simulink model "DDSRFsinglephaseinverter"  (R2023b)
settings: Solver=VariableStepAuto  StartTime=0.0  StopTime=10  RelTol=1e-3
libraries: spsCurrentMeasurementLib x7, spsSeriesRLCBranchLib x7, spsAlphaBetaZerotodq0Lib x4, slpidlib x4, spsIGBTDiodeLib x4, spsVoltageMeasurementLib x4, spsabctoAlphaBetaZeroLib x2, spsdq0toAlphaBetaZeroLib x2, dspinverses x1, spsACVoltageSourceLib x1, spsBreakerLib x1, spsDCVoltageSourceLib x1
settings Model: Creator=Jia Yee Wong  LastModifiedBy=Jia Yee Wong
settings SFSimCC: SimCustomHeaderCode="#include \"ddsrfreferencegen.h\";"  SimUserSources=ddsrfreferencegen.c;

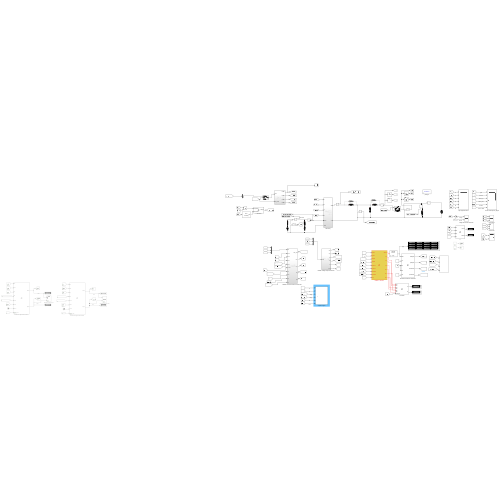
[thumbnail: Simulink's stored preview of the top-level diagram]
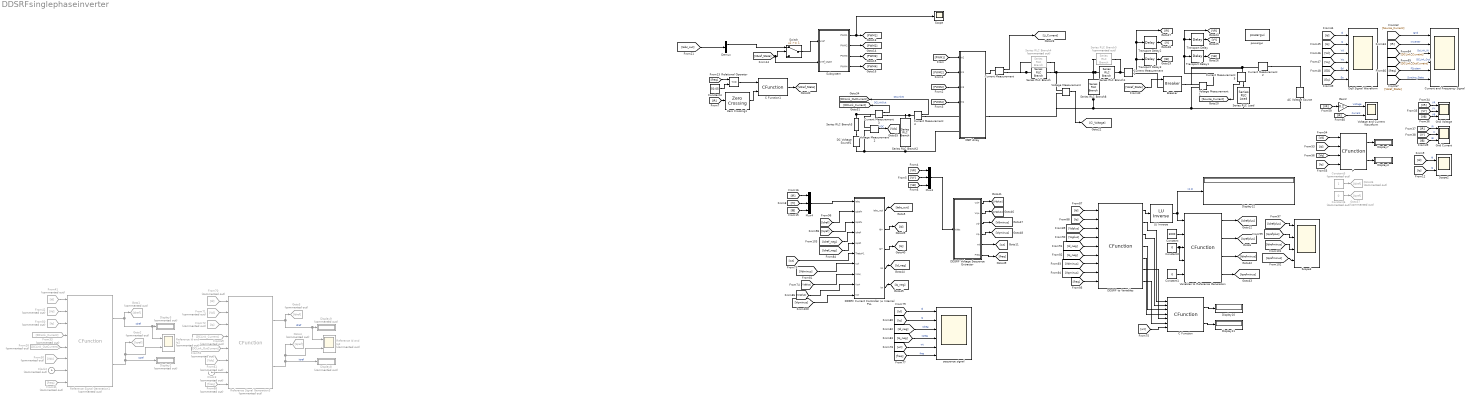
== system DDSRFsinglephaseinverter ==
  " LU Inverse" : dspinverses/ LU Inverse
  AC Voltage Source : spsACVoltageSourceLib/AC Voltage Source  Amplitude=340  Phase=0  Frequency=50  SampleTime=0  Measurements=None  BusType=PV  Pref=100  Qref=100  Qmin=-inf  Qmax=+inf
  Breaker : spsBreakerLib/Breaker  InitialState=0  SwitchingTimes="[1/60  5/60]"  External=on  BreakerResistance=0.00001  SnubberResistance=30  SnubberCapacitance=47e-9  Measurements=None  MoreParameters=on  NoBreakLoop=off
  C Function : CFunction  OutputCode=|
      | P= Po+Pc*cos(2*omegaT)+Ps*sin(2*omegaT);
      | Q= Qo+Qc*cos(2*omegaT)+Qs*sin(2*omegaT);
  C Function1 : CFunction  OutputCode=|  SampleTime=1/50000
      | if(Frequency == true && ZeroCross == 1){
      |     Output = 1;}
      | else if(Frequency == false){
      |         Output = 0;}
  Clock2 : Clock  Commented=on
  Clock3 : Clock  Commented=on
  Constant : Constant  Value=3000
  Constant1 : Constant  Value=0
  Constant2 : Constant  Value=0
  Constant4 : Constant  Value=50.05  SampleTime=1/50000
  Constant5 : Constant  Commented=on
  Constant6 : Constant  Commented=on  Value=0
  Current Measurement{,1..5} (6 alike) : spsCurrentMeasurementLib/Current Measurement  PhasorSimulation=off  OutputType=Complex  PSBequivalent=0
  Current and Frequency Signal : Scope  NumInputPorts=6
  DC Voltage Source1 : spsDCVoltageSourceLib/DC Voltage Source  Amplitude=400  Measurements=None
  DDSRF Current Controller /w Internal PLL : Subsystem
  DDSRF Voltage Sequence Extractor : Subsystem
  DDSRF to Variables : CFunction  OutputCode=|  SampleTime=1/50000
      | if(freq >49.9 && freq <50.1){
      |     Po=(Vdplus*Idplus+Vqplus*Iqplus+Vdminus*Idminus+Vqminus*Iqminus);
      |     Qo=(Vdplus*Idplus-Vqplus*Iqplus+Vdminus*Idminus-Vqminus*Iqminus);
      |     Pc=(Vdminus*Idplus+Vqminus*Iqplus+Vdplus*Iqminus+Vqplus*Iqminus);
      |     Ps=(Vqminus*Idplus-Vdminus*Iqplus-Vqplus*Idminus+Vdplus*Iqminus);
      |     Qc=(Vqminus*Idplus-Vdminus*Iqplus+Vdplus*Idminus-Vdplus*Iqminus);
      |     Qs=(-Vdminus*Idplus-Vqminus*Iqplus+Vdplus*Idminus+Vqplus*Iqminus);
      |     initializeMatrix(matref,Vdplus,Vqplus,Vdminus,Vqminus);
      |     
      |    
      |     }
  Demux : Demux  Outputs=3
  Display{4,7,10..12} (5 alike) : Display
  Display{2..3,8..9} (4 alike) : Display  Commented=on
  Dq0 Signal Waveform : Scope  NumInputPorts=6
  From26 : From  Commented=on  GotoTag=DCLink_OutCurrent
  From30 : From  Commented=on  GotoTag=Vdc
  From31 : From  Commented=on  GotoTag=freq
  From33 : From  Commented=on  GotoTag=DCLink_Current
  From41 : From  Commented=on  GotoTag=Id
  From42 : From  Commented=on  GotoTag=Vd
  From50 : From  Commented=on  GotoTag=Iq
  From51 : From  Commented=on  GotoTag=DCLink_OutCurrent
  From61 : From  Commented=on  GotoTag=Vdc
  From68 : From  Commented=on  GotoTag=freq
  From69 : From  Commented=on  GotoTag=DCLink_Current
  From70 : From  Commented=on  GotoTag=Id
  From71 : From  Commented=on  GotoTag=Vd
  From72 : From  Commented=on  GotoTag=Iq
  Gain2 : Gain  Gain=0.2
  Goto1 : Goto  Commented=on  GotoTag=Idref
  Goto2 : Goto  Commented=on  GotoTag=Iqref
  Goto3 : Goto  Commented=on  GotoTag=Idref
  Goto36 : Goto  Commented=on  GotoTag=Idref
  Goto37 : Goto  Commented=on  GotoTag=Iqref
  Goto4 : Goto  Commented=on  GotoTag=Iqref
  Grid Current : Scope  NumInputPorts=3
  Grid Voltage : Scope  NumInputPorts=3
  IGBT Array : Subsystem
  Mux3 : Mux  Inputs=3
  Mux4 : Mux  Inputs=3
  P : CFunction  OutputCode=|
      | PTotal = Id*Vd;
      | QTotal = Id*Vq-Vq*Id;
  Reference Id and Iq1 : Scope  Commented=on  NumInputPorts=2
  Reference Id and Iq2 : Scope  Commented=on  NumInputPorts=2
  Reference Signal Generation1 : CFunction  Commented=on  OutputCode=|  StartCode=|  SampleTime=1/50000
      OutputCode=|
      | if(Id!=PreviousId || Iq!=PreviousIq){
      |     if(ReferenceGenTrigger(Freq_PLL)){
      |         Idref=IdrefCalc(CLK,Vd,Iin,Iout, Vdc, Vdc);
      |   //Idref =1;
      |    Iqref=0;
      |    PreviousId=Id;
      |    PreviousIq=Iq;
      |    }
      |   
      | } else { Idref = 0; Iqref = 0;}
      StartCode=|
      | PreviousIq =0;
      | PreviousId =0;
  Reference Signal Generation3 : CFunction  Commented=on  OutputCode=|  StartCode=|  SampleTime=1/50000
      OutputCode=|
      | if(Id!=PreviousId || Iq!=PreviousIq){
      |     if(ReferenceGenTrigger(Freq_PLL)){
      |         Idref=IdrefCalc(CLK,Vd,Iin,Iout, Vdc, Vdc);
      |   //Idref =1;
      |    Iqref=0;
      |    PreviousId=Id;
      |    PreviousIq=Iq;
      |    }
      |   
      | } else { Idref = 0; Iqref = 0;}
      StartCode=|
      | PreviousIq =0;
      | PreviousId =0;
  Relational Operator : RelationalOperator  Operator=<=  OutDataTypeStr=boolean  RndMeth=Simplest  InputSameDT=off
  Scope : Scope
  Scope2 : Scope  NumInputPorts=2
  Scope3 : Scope  NumInputPorts=4
  Series RLC Branch : spsSeriesRLCBranchLib/Series RLC Branch  LConnTagsString=__new0  RConnTagsString=__new0  BranchType=L  Resistance=1  Inductance=20.4e-3  SetiL0=off  InitialCurrent=0  Capacitance=1e-6  Setx0=off  InitialVoltage=0  Measurements=None
  Series RLC Branch1 : spsSeriesRLCBranchLib/Series RLC Branch  LConnTagsString=__new0  RConnTagsString=__new0  BranchType=L  Resistance=1  Inductance=148.336e-6  SetiL0=off  InitialCurrent=0  Capacitance=1e-6  Setx0=off  InitialVoltage=0  Measurements=None
  Series RLC Branch2 : spsSeriesRLCBranchLib/Series RLC Branch  LConnTagsString=__new0  RConnTagsString=__new0  BranchType=RC  Resistance=1  Inductance=0  SetiL0=off  InitialCurrent=0  Capacitance=47e-3  Setx0=off  InitialVoltage=300  Measurements=None
  Series RLC Branch3 : spsSeriesRLCBranchLib/Series RLC Branch  LConnTagsString=__new0  RConnTagsString=__new0  BranchType=RL  Resistance=1  Inductance=0  SetiL0=off  InitialCurrent=0  Capacitance=1e-6  Setx0=off  InitialVoltage=0  Measurements=None
  Series RLC Branch4 : spsSeriesRLCBranchLib/Series RLC Branch  Commented=on  LConnTagsString=__new0  RConnTagsString=__new0  BranchType=R  Resistance=220  Inductance=20.4e-3  SetiL0=off  InitialCurrent=0  Capacitance=1e-6  Setx0=off  InitialVoltage=0  Measurements=None
  Series RLC Branch5 : spsSeriesRLCBranchLib/Series RLC Branch  Commented=on  LConnTagsString=__new0  RConnTagsString=__new0  BranchType=R  Resistance=220  Inductance=20.4e-3  SetiL0=off  InitialCurrent=0  Capacitance=1e-6  Setx0=off  InitialVoltage=0  Measurements=None
  Series RLC Branch8 : spsSeriesRLCBranchLib/Series RLC Branch  LConnTagsString=__new0  RConnTagsString=__new0  BranchType=RC  Resistance=120  Inductance=100e-6  SetiL0=off  InitialCurrent=0  Capacitance=5.526e-6  Setx0=off  InitialVoltage=0  Measurements=None
  Series RLC Load : spsSeriesRLCLoadLib/Series RLC Load  LConnTagsString=a  RConnTagsString=__new0  NominalVoltage=240  NominalFrequency=50  ActivePower=10e2  InductivePower=0  CapacitivePower=0  Setx0=off  InitialVoltage=240  SetiL0=off  InitialCurrent=10  Measurements=None  LoadType=constant PQ
  Subsystem : Subsystem
  Switch : Switch  Threshold=1  SaturateOnIntegerOverflow=off  InputSameDT=off
  Transport Delay : TransportDelay  DelayTime=6.67e-3  BufferSize=4096
  Transport Delay1 : TransportDelay  DelayTime=13.34e-3  BufferSize=5120
  Transport Delay2 : TransportDelay  DelayTime=6.67e-3  BufferSize=4096
  Transport Delay3 : TransportDelay  DelayTime=13.34e-3  BufferSize=4096
  Variables to Reference Generation : CFunction  OutputCode=|
      | Idrefplus = mat[0][0] * Po + mat[0][1] * 0 + mat[0][2] * 0 + mat[0][3] * Qo;
      | Iqrefplus = mat[1][0] * Po + mat[1][1] * 0 + mat[1][2] * 0 + mat[1][3] * Qo;
      | Idrefminus = mat[2][0] * Po - mat[2][1] * 0 - mat[2][2] * 0 + mat[2][3] * Qo;
      | Iqrefminus = mat[3][0] * Po - mat[3][1] * 0 + mat[3][2] * 0 - mat[3][3] * Qo;
  Voltage Measurement : spsVoltageMeasurementLib/Voltage Measurement  PhasorSimulation=off  OutputType=Complex  PSBequivalent=0
  Voltage Measurement1 : spsVoltageMeasurementLib/Voltage Measurement  PhasorSimulation=off  OutputType=Complex  PSBequivalent=0
  Voltage Measurement2 : spsVoltageMeasurementLib/Voltage Measurement  PhasorSimulation=off  OutputType=Complex  PSBequivalent=0
  Voltage and Current Waveform : Scope  NumInputPorts=2
  Zero Crossing1 : dspsigops/Zero Crossing
  powergui : spspowerguiLib/powergui  Priority=1  SimulationMode=Continuous  SampleTime=50e-6  frequency=60  Iterations=50  frequencyindice=0  Pbase=100e6  ErrMax=1e-4  UnitsV=kV  UnitsW=MW  buscounter=0  FunctionMessages=off  echomessages=off  EnableUseOfTLC=off  CurrentSourceSwitches=off  DisableSnubberDevices=off  DisableRonSwitches=off  DisableVfSwitches=off  DisplayEquations=off  AutomaticDiscreteSolvers=off  SolverType=Tustin/Backward Euler (TBE)  Interpol=off  ExternalGateDelay=off  methode=off  Ts=100  x0status=blocks  SPID=on  SwTol=0  HookPort=off  NonlinearTolerance=1e-4  nMaxIteration=100  ContinueOnMaxIteration=off  RestoreLinks=warning  ResistiveCurrentMeasurement=off  Frange=[0:2:500]  Ylog=off  Xlog=on  ShowGrid=off  save=off  variable=ZData  structure=0  ZoomFFT=off  StartTime=0.0  cycles=1  DisplayStyle=1  fundamental=60  FreqAxis=off  MaxFrequency=1000  frequencyindicesteady=1  RmsSteady=1  display=off
  sequence signal : Scope  NumInputPorts=6
  wires:
  [IR] -> Voltage and Current Waveform/2  "Current"
  [Iq] -> P/4
  Subsystem/4(PWM4) -> [PWM4]
  Switch/1 -> Subsystem/1(Vref)
  Constant5/1 -> Goto36/1
  [Id] -> P/2
  Current Measurement3/1 -> [DCLink_Current]  "DCLinkOut"
  Transport Delay3/1 -> [IB]
  [VY] -> Grid Voltage/2  "VY"
  [IY] -> Grid Current/2  "IY"
  Subsystem/1(PWM1) -> Scope/1, [PWM1]
  [VR] -> Grid Voltage/1  "VR"
  Demux/1 -> Switch/1
  [freq] -> Relational Operator/1
  Constant4/1 -> Relational Operator/2
  [VB] -> Grid Voltage/3  "VB"
  Subsystem/2(PWM2) -> [PWM2]
  Current Measurement/1 -> [Li_Current]
  Transport Delay1/1 -> [VB]
  Transport Delay2/1 -> [IY]
  Transport Delay/1 -> [VY]
  [VAref_State] -> Breaker/1
  [VR] -> Gain2/1
  Relational Operator/1 -> C Function1/1
  [IR] -> Current and Frequency Signal/2  "Iinverter"
  [Id] -> Scope2/1  "Id"
  Constant6/1 -> Goto37/1
  [Vd] -> Dq0 Signal Waveform/3  "Vd"
  C Function1/1 -> [VAref_State]
  Zero Crossing1/1 -> C Function1/2
  Current Measurement4/1 -> [DCLink_OutCurrent]  "DCLinkIN"
  [IR] -> Zero Crossing1/1
  [Source_Current] -> Current and Frequency Signal/1  "Igrid"
  [VAref_State] -> Current and Frequency Signal/6  "Synchro_State"
  Voltage Measurement2/1 -> [Vdc]  "VDC"
  Current Measurement1/1 -> [IR], Transport Delay2/1, Transport Delay3/1
  Gain2/1 -> Voltage and Current Waveform/1  "Voltage"
  [Vq] -> Dq0 Signal Waveform/4  "Vq"
  Subsystem/3(PWM3) -> [PWM3]
  [IB] -> Grid Current/3  "IB"
  [DCLink_OutCurrent] -> Current and Frequency Signal/4  "DCLink_Out"
  [PWM2] -> IGBT Array/2(In1)
  [DCLink_Current] -> Current and Frequency Signal/3  "DcLink_IN"
  [PWM3] -> IGBT Array/3(In3)
  [ED] -> Dq0 Signal Waveform/5  "Ed"
  Voltage Measurement1/1 -> [VR], Transport Delay/1, Transport Delay1/1
  P/1 -> Display7/1
  [IR] -> Grid Current/1  "IR"
  [Vq] -> P/3
  [PWM1] -> IGBT Array/1(In2)
  [Vd] -> P/1
  P/2 -> Display4/1
  [PWM4] -> IGBT Array/4(In4)
  Voltage Measurement/1 -> [Ci_Voltage]
  Current Measurement5/1 -> [Source_Current]
  [freq] -> Current and Frequency Signal/5  "FSystem"
  [Id] -> Dq0 Signal Waveform/1  "Id"
  [Iq] -> Dq0 Signal Waveform/2  "Iq"
  [Eq] -> Dq0 Signal Waveform/6  "Eq"
  [Iq] -> Scope2/2  "Iq"
  [VAref_State] -> Subsystem/2(Vref_state), Switch/2
  Reference Signal Generation1/1 -> Reference Id and Iq1/1, Display3/1, Goto1/1  "Idref"
  From26/1 -> Reference Signal Generation1/5
  From42/1 -> Reference Signal Generation1/2
  From50/1 -> Reference Signal Generation1/3
  From31/1 -> Reference Signal Generation1/8
  Reference Signal Generation1/2 -> Reference Id and Iq1/2, Goto2/1, Display2/1  "Iqref"
  Clock2/1 -> Reference Signal Generation1/7
  From30/1 -> Reference Signal Generation1/6
  From33/1 -> Reference Signal Generation1/4
  From41/1 -> Reference Signal Generation1/1
  From70/1 -> Reference Signal Generation3/1
  Clock3/1 -> Reference Signal Generation3/7
  From69/1 -> Reference Signal Generation3/4
  Reference Signal Generation3/2 -> Reference Id and Iq2/2, Goto4/1, Display8/1  "Iqref"
  From68/1 -> Reference Signal Generation3/8
  From61/1 -> Reference Signal Generation3/6
  From72/1 -> Reference Signal Generation3/3
  From71/1 -> Reference Signal Generation3/2
  From51/1 -> Reference Signal Generation3/5
  Reference Signal Generation3/1 -> Reference Id and Iq2/1, Display9/1, Goto3/1  "Idref"
  DDSRF to Variables/2 -> C Function/1
  C Function/1 -> Display10/1
  DDSRF to Variables/3 -> C Function/2
  [Vdplus] -> DDSRF Current Controller /w Internal PLL/8(Vd+\)
  C Function/2 -> Display11/1
  " LU Inverse"/1 -> Variables to Reference Generation/1, Display12/1  "[4 4]"
  [Id] -> sequence signal/1  "Id"
  [Id_neg] -> sequence signal/3  "Idneg"
  DDSRF to Variables/6 -> C Function/5
  [wt] -> DDSRF Current Controller /w Internal PLL/6(Theta*1)
  Constant1/1 -> Variables to Reference Generation/5
  Constant/1 -> Variables to Reference Generation/2
  [wt] -> sequence signal/5  "wt"
  [Iq_neg] -> sequence signal/4  "iqneg"
  DDSRF Voltage Sequence Extractor/5(wt) -> [wt]
  [Iq] -> sequence signal/2  "Iq"
  [Vqplus] -> DDSRF Current Controller /w Internal PLL/9(Vq+)
  [Vdminus] -> DDSRF Current Controller /w Internal PLL/7(Vd-)
  [Iqrefplus] -> Scope3/2
  [Idref_neg] -> DDSRF Current Controller /w Internal PLL/5(Iqref-)
  Variables to Reference Generation/2 -> [Iqrefplus]
  Variables to Reference Generation/1 -> [Idrefplus]
  [Vdminus] -> DDSRF to Variables/7
  [Vqminus] -> DDSRF Current Controller /w Internal PLL/10(Vq-)
  DDSRF Voltage Sequence Extractor/3(Vd-) -> [Vdminus]
  [Id_neg] -> DDSRF to Variables/5
  [Iqref] -> DDSRF Current Controller /w Internal PLL/3(Iqref+)
  [Idrefplus] -> Scope3/1
  [wt] -> C Function/7
  DDSRF to Variables/5 -> C Function/4
  [Iq_neg] -> DDSRF to Variables/6
  [Idrefminus] -> Scope3/3
  [Vdplus] -> DDSRF to Variables/3
  DDSRF Voltage Sequence Extractor/4(Vq-) -> [Vqminus]
  DDSRF Current Controller /w Internal PLL/3(Iq+) -> [Iq]
  Variables to Reference Generation/4 -> [Iqrefminus]
  [freq] -> sequence signal/6  "freq"
  [Id] -> DDSRF to Variables/1
  DDSRF Voltage Sequence Extractor/6(Freq) -> [freq]
  [Vqminus] -> DDSRF to Variables/8
  DDSRF to Variables/1 -> " LU Inverse"/1
  [freq] -> DDSRF to Variables/9
  Variables to Reference Generation/3 -> [Idrefminus]
  [Iqrefminus] -> Scope3/4
  DDSRF to Variables/7 -> C Function/6
  [Vqplus] -> DDSRF to Variables/4
  DDSRF Voltage Sequence Extractor/2(Vq+) -> [Vqplus]
  [Iq] -> DDSRF to Variables/2
  DDSRF Voltage Sequence Extractor/1(Vd+) -> [Vdplus]
  DDSRF Current Controller /w Internal PLL/1(Iabc_out) -> [Iabc_out]
  DDSRF Current Controller /w Internal PLL/2(Id+) -> [Id]
  [Idref_neg] -> DDSRF Current Controller /w Internal PLL/4(Idref-)
  DDSRF Current Controller /w Internal PLL/5(Iq-) -> [Iq_neg]
  DDSRF to Variables/4 -> C Function/3
  [Idref] -> DDSRF Current Controller /w Internal PLL/2(Idref+)
  DDSRF Current Controller /w Internal PLL/4(Id-) -> [Id_neg]
  Mux3/1 -> DDSRF Voltage Sequence Extractor/1(Vabc)
  [VB] -> Mux3/3
  [VR] -> Mux3/1
  [VY] -> Mux3/2
  Mux4/1 -> DDSRF Current Controller /w Internal PLL/1(Iabc)
  [IY] -> Mux4/2
  [IB] -> Mux4/3
  [IR] -> Mux4/1
  [Iabc_out] -> Demux/1
  Constant2/1 -> Variables to Reference Generation/4, Variables to Reference Generation/3
  connections:
  Current Measurement4/LConn1 -- Current Measurement3/RConn1 -- Series RLC Branch2/LConn1
  Series RLC Branch8/RConn1 -- IGBT Array/RConn2 -- Voltage Measurement/LConn2 -- AC Voltage Source/LConn1 -- Series RLC Load/RConn1 -- Voltage Measurement1/LConn2
  Voltage Measurement2/LConn2 -- Series RLC Branch2/RConn1 -- IGBT Array/LConn2 -- DC Voltage Source1/LConn1
  Series RLC Branch1/LConn1 -- Series RLC Branch8/LConn1 -- Series RLC Branch5/LConn1 -- Voltage Measurement/LConn1 -- Series RLC Branch/RConn1 -- Series RLC Branch4/RConn1
  Series RLC Branch3/LConn1 -- Current Measurement3/LConn1 -- Voltage Measurement2/LConn1
  Current Measurement1/LConn1 -- Series RLC Branch5/RConn1 -- Series RLC Branch1/RConn1
  Current Measurement2/RConn1 -- Breaker/RConn1 -- Voltage Measurement1/LConn1 -- Current Measurement5/LConn1
  Series RLC Branch/LConn1 -- Current Measurement/RConn1 -- Series RLC Branch4/LConn1
  IGBT Array/RConn1 -- Current Measurement/LConn1
  Current Measurement4/RConn1 -- IGBT Array/LConn1
  Breaker/LConn1 -- Current Measurement1/RConn1
  Current Measurement2/LConn1 -- AC Voltage Source/RConn1
  Current Measurement5/RConn1 -- Series RLC Load/LConn1
  Series RLC Branch3/RConn1 -- DC Voltage Source1/RConn1

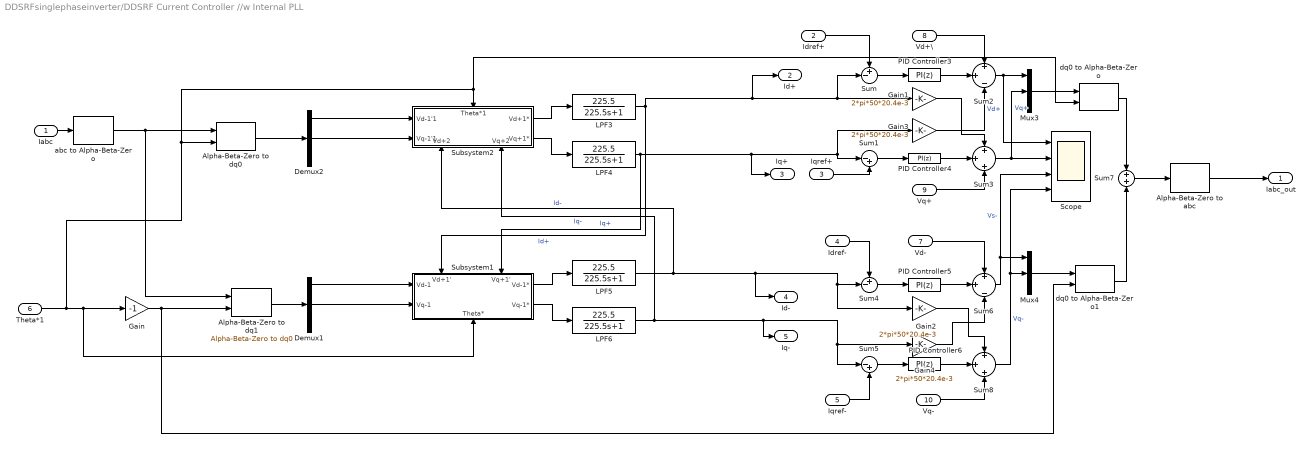
== system DDSRFsinglephaseinverter/DDSRF Current Controller //w Internal PLL ==
  Iabc : Inport
  Idref+ : Inport  Port=2
  Iqref+ : Inport  Port=3
  Idref- : Inport  Port=4
  Iqref- : Inport  Port=5
  Theta*1 : Inport  Port=6
  Vd- : Inport  Port=7
  Vd+\ : Inport  Port=8
  Vq+ : Inport  Port=9
  Vq- : Inport  Port=10
  Alpha-Beta-Zero to abc : spsAlphaBetaZerotoabcLib/Alpha-Beta-Zero to abc
      settings: LibrarySourceBlock=|
      | sps_lib/Control/Alpha-Beta-Zero
      | to abc
  Alpha-Beta-Zero to dq0 : spsAlphaBetaZerotodq0Lib/Alpha-Beta-Zero to dq0  Alignment=90 degrees behind phase A axis
  Alpha-Beta-Zero to dq1 : spsAlphaBetaZerotodq0Lib/Alpha-Beta-Zero to dq0  Alignment=90 degrees behind phase A axis
  Demux1 : Demux  Outputs=3
  Demux2 : Demux  Outputs=3
  Gain : Gain  Gain=-1
  Gain{1..4} (4 alike) : Gain  Gain=2*pi*50*20.4e-3
  LPF{3..6} (4 alike) : TransferFcn  Numerator=[225.5]  Denominator=[225.5 1]
  Mux3 : Mux  Inputs=3
  Mux4 : Mux  Inputs=3
  PID Controller{3..6} (4 alike) : slpidlib/PID Controller  Controller=PI  Form=Parallel  TimeDomain=Discrete-time  UseExternalTs=off  SampleTime=1/50000  IntegratorMethod=Forward Euler  FilterMethod=Forward Euler  ControllerParametersSource=internal  P=0.5  I=0.02  UseKiTs=off  D=0  N=100  UseFilter=on  TunerSelectOption=Transfer Function Based (PID Tuner App)  InitialConditionSource=internal  InitialConditionForIntegrator=0  InitialConditionForFilter=0  DifferentiatorICPrevScaledInput=0  ExternalReset=none  TrackingMode=off  Kt=1  LimitOutput=off  SatLimitsSource=internal  UpperSaturationLimit=inf  LowerSaturationLimit=-inf  LinearizeAsGain=on  AntiWindupMode=none  Kb=1  LimitIntegrator=off  UpperIntegratorSaturationLimit=inf  LowerIntegratorSaturationLimit=-inf  POutMin=[]  POutMax=[]  IOutMin=[]  IOutMax=[]  DOutMin=[]  DOutMax=[]  NOutMin=[]  NOutMax=[]  SumOutMin=[]  SumOutMax=[]  SaturationOutMin=[]  SaturationOutMax=[]  PParamMin=[]  PParamMax=[]  IParamMin=[]  IParamMax=[]  DParamMin=[]  DParamMax=[]  NParamMin=[]  NParamMax=[]  KbParamMin=[]  KbParamMax=[]  KtParamMin=[]  KtParamMax=[]  KbOutMin=[]  KbOutMax=[]  KtOutMin=[]  KtOutMax=[]  IntegratorOutMin=[]  IntegratorOutMax=[]  FilterOutMin=[]  FilterOutMax=[]  SumI1OutMin=[]  SumI1OutMax=[]  SumI2OutMin=[]  SumI2OutMax=[]  SumI3OutMin=[]  SumI3OutMax=[]  SumI4OutMin=[]  SumI4OutMax=[]  SumDOutMin=[]  SumDOutMax=[]  DifferentiatorOutMin=[]  DifferentiatorOutMax=[]  FilterDiffOutCoefMin=[]  FilterDiffOutCoefMax=[]  ReciprocalOutMin=[]  ReciprocalOutMax=[]  SumDenOutMin=[]  SumDenOutMax=[]  SumNumOutMin=[]  SumNumOutMax=[]  DivideOutMin=[]  DivideOutMax=[]  UdiffTsProdOutMin=[]  UdiffTsProdOutMax=[]  NTsProdOutMin=[]  NTsProdOutMax=[]  UintegralTsProdOutMin=[]  UintegralTsProdOutMax=[]  UngainTsProdOutMin=[]  UngainTsProdOutMax=[]  ClampingZeroOutDataTypeStr=Inherit: Inherit via back propagation  ClampingZeroOutMin=[]  ClampingZeroOutMax=[]  FilterDenConstantOutDataTypeStr=Inherit: Inherit via back propagation  FilterDenConstantOutMin=[]  FilterDenConstantOutMax=[]  PCopyOutDataTypeStr=Inherit: Inherit via back propagation  PCopyOutMin=[]  PCopyOutMax=[]  NCopyOutDataTypeStr=Inherit: Inherit via back propagation  NCopyOutMin=[]  NCopyOutMax=[]  IntegratorContinuousStateAttributes=''  IntegratorStateMustResolveToSignalObject=off  IntegratorRTWStateStorageClass=Auto  FilterContinuousStateAttributes=''  FilterStateMustResolveToSignalObject=off  FilterRTWStateStorageClass=Auto  ParallelPVariant=InternalParameters  IdealPVariant=Disabled  IVariant=InternalParameters  DVariant=Disabled  IntegratorVariant=Discrete  SatVariant=Disabled  AWVariant=Passthrough  PCopyVariant=Disabled  TRVariant=Disabled  FdbkBlocksVariant=Forward  IdealPFdbkVariant=Disabled  SatFdbkVariant=Disabled  DerivativeFilterVariant=Disabled  NVariant=Disabled  NCopyVariant=Disabled_SignalSpec  FilterICVariant=Disabled  IntegratorICVariant=InternalICs  ExternalResetVariant=Disabled  TRSumVariant=Passthrough  SumFdbkVariant=Disabled  SumVariant=Sum_PI  TsampFilterVariant=InternalTs  TsampNgainVariant=Passthrough  TsampIntegralVariant=Disabled_SignalSpec  ExternalSaturationOutDataTypeStr=Inherit: Same as second input
  Scope : Scope  NumInputPorts=4
  Subsystem1 : Subsystem
      settings: PortSchema="{\"entries\":[{\"content\":{\"sides\":[{\"content\":{\"connectorIds\":[\"In1\",\"In2\"]},\"type\":\"ConnectorPlacement.EquallySpacedRectSide\",\"uuid\":\"90520742-b67b-401b-a323-e780c78b1482\"},{\"content\":{\"connectorIds\":[\"Out1\",\"Out2\"],\"side\":\"RIGHT\"},\"type\":\"ConnectorPlacement.EquallySpacedRectSide\",\"uuid\":\"13b71677-6011-49b4-a8e2-8815d9fe4fc1\"},{\"content\":{\"connectorIds\":[\"In3\",\"In4\"],\"side\":\"TOP\"},\"type\":\"ConnectorPlacement.EquallySpacedRectSide\",\"uuid\":\"b0f32480-838e-4ed7-8c04-14ce7fe710af\"},{\"content\":{\"connectorIds\":[\"In5\"],\"side\":\"BOTTOM\"},\"type\":\"ConnectorPlacement.EquallySpacedRectSide\",\"uuid\":\"11e8df11-2f01-47a5-9567-d29a5352b573\"}]},\"type\":\"ConnectorPlacement.EquallySpacedConnector\",\"uuid\":\"d99c7ffd-2341-4980-bdb2-3a875f1b77ee\"}],\"packageUris\":[\"http://schema.mathworks.com/mf0/Connector/R2020b\"],\"version\":\"1.0\"}"
  Subsystem2 : Subsystem
      settings: PortSchema="{\"entries\":[{\"content\":{\"sides\":[{\"content\":{\"connectorIds\":[\"In1\",\"In2\"]},\"type\":\"ConnectorPlacement.EquallySpacedRectSide\",\"uuid\":\"90520742-b67b-401b-a323-e780c78b1482\"},{\"content\":{\"connectorIds\":[\"Out1\",\"Out2\"],\"side\":\"RIGHT\"},\"type\":\"ConnectorPlacement.EquallySpacedRectSide\",\"uuid\":\"13b71677-6011-49b4-a8e2-8815d9fe4fc1\"},{\"content\":{\"connectorIds\":[\"In3\"],\"side\":\"TOP\"},\"type\":\"ConnectorPlacement.EquallySpacedRectSide\",\"uuid\":\"b0f32480-838e-4ed7-8c04-14ce7fe710af\"},{\"content\":{\"connectorIds\":[\"In4\",\"In5\"],\"side\":\"BOTTOM\"},\"type\":\"ConnectorPlacement.EquallySpacedRectSide\",\"uuid\":\"7441e455-6112-4477-b61e-4bb135ec9e12\"}]},\"type\":\"ConnectorPlacement.EquallySpacedConnector\",\"uuid\":\"d99c7ffd-2341-4980-bdb2-3a875f1b77ee\"}],\"packageUris\":[\"http://schema.mathworks.com/mf0/Connector/R2020b\"],\"version\":\"1.0\"}"
  Sum : Sum  Inputs=+-|
  Sum1 : Sum  Inputs=|-+
  Sum2 : Sum  Inputs=+|+|-
  Sum3 : Sum  Inputs=+|+|+
  Sum4 : Sum  Inputs=+-|
  Sum5 : Sum  Inputs=|-+
  Sum6 : Sum  Inputs=+|+|-
  Sum7 : Sum  Inputs=+|+
  Sum8 : Sum  Inputs=+|+|+
  abc to Alpha-Beta-Zero : spsabctoAlphaBetaZeroLib/abc to Alpha-Beta-Zero
  dq0 to Alpha-Beta-Zero : spsdq0toAlphaBetaZeroLib/dq0 to Alpha-Beta-Zero  Alignment=90 degrees behind phase A axis
  dq0 to Alpha-Beta-Zero1 : spsdq0toAlphaBetaZeroLib/dq0 to Alpha-Beta-Zero  Alignment=90 degrees behind phase A axis
  Iabc_out : Outport
  Id+ : Outport  Port=2
  Iq+ : Outport  Port=3
  Id- : Outport  Port=4
  Iq- : Outport  Port=5
  wires:
  Mux3/1 -> dq0 to Alpha-Beta-Zero/1
  Gain2/1 -> Sum8/1
  Sum8/1 -> Scope/4, Mux4/2  "Vq-"
  LPF5/1 -> Gain2/1, Sum4/2, Id-/1, Subsystem2/4(Vd+2)  "Id-"
  Iabc/1 -> abc to Alpha-Beta-Zero/1
  Mux4/1 -> dq0 to Alpha-Beta-Zero1/1
  Idref-/1 -> Sum4/1
  Sum6/1 -> Scope/3, Mux4/1  "Vs-"
  LPF6/1 -> Iq-/1, Gain4/1, Sum5/1, Subsystem2/5(Vq+2)  "Iq-"
  Demux2/2 -> Subsystem2/2(Vq-1'1)
  Idref+/1 -> Sum/1
  Iqref+/1 -> Sum1/2
  dq0 to Alpha-Beta-Zero/1 -> Sum7/1
  LPF4/1 -> Subsystem1/4(Vq+1'), Iq+/1, Gain3/1, Sum1/1  "Iq+"
  Sum5/1 -> PID Controller6/1
  Sum/1 -> PID Controller3/1
  Subsystem2/1(Vd+1*) -> LPF3/1
  Demux2/1 -> Subsystem2/1(Vd-1'1)
  Subsystem1/2(Vq-1*) -> LPF6/1
  Sum1/1 -> PID Controller4/1
  dq0 to Alpha-Beta-Zero1/1 -> Sum7/2
  Iqref-/1 -> Sum5/2
  LPF3/1 -> Id+/1, Gain1/1, Sum/2, Subsystem1/3(Vd+1')  "Id+"
  Gain1/1 -> Sum3/1
  PID Controller6/1 -> Sum8/2
  Sum4/1 -> PID Controller5/1
  Sum3/1 -> Scope/2, Mux3/2  "Vq+"
  Subsystem1/1(Vd-1*) -> LPF5/1
  PID Controller4/1 -> Sum3/2
  Subsystem2/2(Vq+1*) -> LPF4/1
  Alpha-Beta-Zero to dq0/1 -> Demux2/1
  abc to Alpha-Beta-Zero/1 -> Alpha-Beta-Zero to dq0/1, Alpha-Beta-Zero to dq1/1
  Demux1/1 -> Subsystem1/1(Vd-1)
  Alpha-Beta-Zero to dq1/1 -> Demux1/1
  Gain/1 -> dq0 to Alpha-Beta-Zero1/2, Alpha-Beta-Zero to dq1/2
  Sum2/1 -> Scope/1, Mux3/1  "Vd+"
  Demux1/2 -> Subsystem1/2(Vq-1)
  Sum7/1 -> Alpha-Beta-Zero to abc/1
  Alpha-Beta-Zero to abc/1 -> Iabc_out/1
  Theta*1/1 -> Subsystem1/5(Theta*), Gain/1, Subsystem2/3(Theta*1), dq0 to Alpha-Beta-Zero/2, Alpha-Beta-Zero to dq0/2
  PID Controller3/1 -> Sum2/2
  Gain3/1 -> Sum2/3
  Gain4/1 -> Sum6/3
  PID Controller5/1 -> Sum6/2
  Vd-/1 -> Sum6/1
  Vd+\/1 -> Sum2/1
  Vq+/1 -> Sum3/3
  Vq-/1 -> Sum8/3

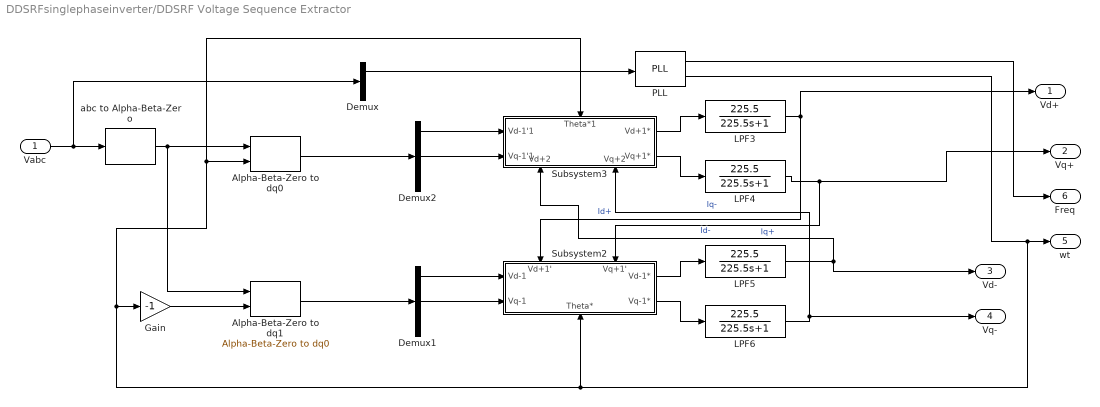
== system DDSRFsinglephaseinverter/DDSRF Voltage Sequence Extractor ==
  Vabc : Inport
  Alpha-Beta-Zero to dq0 : spsAlphaBetaZerotodq0Lib/Alpha-Beta-Zero to dq0  Alignment=90 degrees behind phase A axis
  Alpha-Beta-Zero to dq1 : spsAlphaBetaZerotodq0Lib/Alpha-Beta-Zero to dq0  Alignment=90 degrees behind phase A axis
  Demux : Demux  Outputs=3
  Demux1 : Demux  Outputs=3
  Demux2 : Demux  Outputs=3
  Gain : Gain  Gain=-1
  LPF{3..6} (4 alike) : TransferFcn  Numerator=[225.5]  Denominator=[225.5 1]
  PLL : spsPLLLib/PLL  Fmin=45  Par_Init=[0, 60]  ParK=[180, 3200, 1]  TcD=1e-4  MaxRateChangeFreq=12  FilterCutOffFreq=25  Ts=0  AGC=on
      settings: LibrarySourceBlock=sps_lib/Control/PLL
  Subsystem2 : Subsystem
      settings: PortSchema="{\"entries\":[{\"content\":{\"sides\":[{\"content\":{\"connectorIds\":[\"In1\",\"In2\"]},\"type\":\"ConnectorPlacement.EquallySpacedRectSide\",\"uuid\":\"90520742-b67b-401b-a323-e780c78b1482\"},{\"content\":{\"connectorIds\":[\"Out1\",\"Out2\"],\"side\":\"RIGHT\"},\"type\":\"ConnectorPlacement.EquallySpacedRectSide\",\"uuid\":\"13b71677-6011-49b4-a8e2-8815d9fe4fc1\"},{\"content\":{\"connectorIds\":[\"In3\",\"In4\"],\"side\":\"TOP\"},\"type\":\"ConnectorPlacement.EquallySpacedRectSide\",\"uuid\":\"b0f32480-838e-4ed7-8c04-14ce7fe710af\"},{\"content\":{\"connectorIds\":[\"In5\"],\"side\":\"BOTTOM\"},\"type\":\"ConnectorPlacement.EquallySpacedRectSide\",\"uuid\":\"11e8df11-2f01-47a5-9567-d29a5352b573\"}]},\"type\":\"ConnectorPlacement.EquallySpacedConnector\",\"uuid\":\"d99c7ffd-2341-4980-bdb2-3a875f1b77ee\"}],\"packageUris\":[\"http://schema.mathworks.com/mf0/Connector/R2020b\"],\"version\":\"1.0\"}"
  Subsystem3 : Subsystem
      settings: PortSchema="{\"entries\":[{\"content\":{\"sides\":[{\"content\":{\"connectorIds\":[\"In1\",\"In2\"]},\"type\":\"ConnectorPlacement.EquallySpacedRectSide\",\"uuid\":\"90520742-b67b-401b-a323-e780c78b1482\"},{\"content\":{\"connectorIds\":[\"Out1\",\"Out2\"],\"side\":\"RIGHT\"},\"type\":\"ConnectorPlacement.EquallySpacedRectSide\",\"uuid\":\"13b71677-6011-49b4-a8e2-8815d9fe4fc1\"},{\"content\":{\"connectorIds\":[\"In3\"],\"side\":\"TOP\"},\"type\":\"ConnectorPlacement.EquallySpacedRectSide\",\"uuid\":\"b0f32480-838e-4ed7-8c04-14ce7fe710af\"},{\"content\":{\"connectorIds\":[\"In4\",\"In5\"],\"side\":\"BOTTOM\"},\"type\":\"ConnectorPlacement.EquallySpacedRectSide\",\"uuid\":\"7441e455-6112-4477-b61e-4bb135ec9e12\"}]},\"type\":\"ConnectorPlacement.EquallySpacedConnector\",\"uuid\":\"d99c7ffd-2341-4980-bdb2-3a875f1b77ee\"}],\"packageUris\":[\"http://schema.mathworks.com/mf0/Connector/R2020b\"],\"version\":\"1.0\"}"
  abc to Alpha-Beta-Zero : spsabctoAlphaBetaZeroLib/abc to Alpha-Beta-Zero
  Vd+ : Outport
  Vq+ : Outport  Port=2
  Vd- : Outport  Port=3
  Vq- : Outport  Port=4
  wt : Outport  Port=5
  Freq : Outport  Port=6
  wires:
  Demux2/1 -> Subsystem3/1(Vd-1'1)
  Subsystem2/1(Vd-1*) -> LPF5/1
  LPF5/1 -> Vd-/1, Subsystem3/4(Vd+2)  "Id-"
  LPF4/1 -> Subsystem2/4(Vq+1'), Vq+/1  "Iq+"
  LPF6/1 -> Vq-/1, Subsystem3/5(Vq+2)  "Iq-"
  LPF3/1 -> Vd+/1, Subsystem2/3(Vd+1')  "Id+"
  Subsystem2/2(Vq-1*) -> LPF6/1
  Demux2/2 -> Subsystem3/2(Vq-1'1)
  Alpha-Beta-Zero to dq0/1 -> Demux2/1
  abc to Alpha-Beta-Zero/1 -> Alpha-Beta-Zero to dq1/1, Alpha-Beta-Zero to dq0/1
  Alpha-Beta-Zero to dq1/1 -> Demux1/1
  Demux1/1 -> Subsystem2/1(Vd-1)
  Demux1/2 -> Subsystem2/2(Vq-1)
  Gain/1 -> Alpha-Beta-Zero to dq1/2
  Vabc/1 -> Demux/1, abc to Alpha-Beta-Zero/1
  Subsystem3/1(Vd+1*) -> LPF3/1
  Subsystem3/2(Vq+1*) -> LPF4/1
  Demux/1 -> PLL/1
  PLL/2 -> Subsystem2/5(Theta*), Subsystem3/3(Theta*1), Alpha-Beta-Zero to dq0/2, Gain/1, wt/1
  PLL/1 -> Freq/1

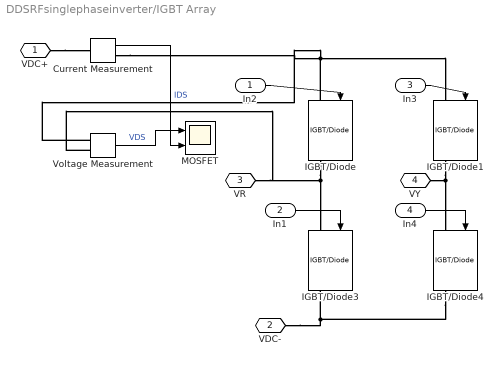
== system DDSRFsinglephaseinverter/IGBT Array ==
  In2 : Inport
  In1 : Inport  Port=2
  In3 : Inport  Port=3
  In4 : Inport  Port=4
  Current Measurement : spsCurrentMeasurementLib/Current Measurement  PhasorSimulation=off  OutputType=Complex  PSBequivalent=0
  IGBT/Diode{,1,3..4} (4 alike) : spsIGBTDiodeLib/IGBT//Diode  Ron=1e-3  Rs=1e5  Cs=inf  Measurements=on
  MOSFET : Scope  NumInputPorts=2
  Voltage Measurement : spsVoltageMeasurementLib/Voltage Measurement  PhasorSimulation=off  OutputType=Complex  PSBequivalent=0
  VDC+ : PMIOPort  Side=Left
  VDC- : PMIOPort  Port=2  Side=Left
  VR : PMIOPort  Port=3  Side=Right
  VY : PMIOPort  Port=4  Side=Right
  wires:
  In1/1 -> IGBT/Diode3/1
  In4/1 -> IGBT/Diode4/1
  In3/1 -> IGBT/Diode1/1
  In2/1 -> IGBT/Diode/1
  Voltage Measurement/1 -> MOSFET/1  "VDS"
  Current Measurement/1 -> MOSFET/2  "IDS"
  connections:
  IGBT/Diode4/RConn1 -- VDC-/RConn1 -- IGBT/Diode3/RConn1
  IGBT/Diode/RConn1 -- Voltage Measurement/LConn2 -- VR/RConn1 -- IGBT/Diode3/LConn1
  IGBT/Diode1/RConn1 -- VY/RConn1 -- IGBT/Diode4/LConn1
  IGBT/Diode/LConn1 -- Current Measurement/RConn1 -- Voltage Measurement/LConn1 -- IGBT/Diode1/LConn1
  VDC+/RConn1 -- Current Measurement/LConn1

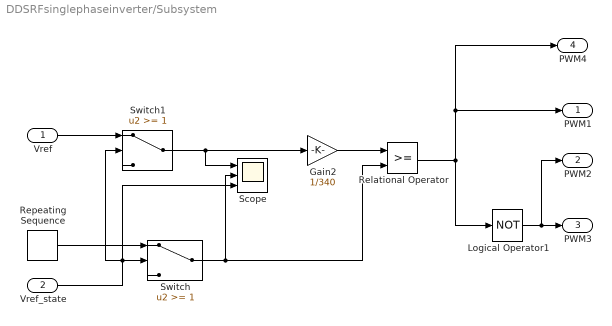
== system DDSRFsinglephaseinverter/Subsystem ==
  Vref : Inport
  Vref_state : Inport  Port=2
  Gain2 : Gain  Gain=1/340
  Logical Operator1 : Logic  Operator=NOT  AllPortsSameDT=off  OutDataTypeStr=boolean
  Relational Operator : RelationalOperator  OutDataTypeStr=boolean  RndMeth=Simplest  InputSameDT=off
  Repeating Sequence : simulink/Sources/Repeating Sequence  rep_seq_t=[0 0.00005 0.0001]  rep_seq_y=[-1 1 -1]
  Scope : Scope  NumInputPorts=3
  Switch : Switch  Threshold=1  SaturateOnIntegerOverflow=off  InputSameDT=off
  Switch1 : Switch  Threshold=1  SaturateOnIntegerOverflow=off  InputSameDT=off
  PWM1 : Outport
  PWM2 : Outport  Port=2
  PWM3 : Outport  Port=3
  PWM4 : Outport  Port=4
  wires:
  Gain2/1 -> Relational Operator/1
  Relational Operator/1 -> Logical Operator1/1, PWM1/1, PWM4/1
  Logical Operator1/1 -> PWM2/1, PWM3/1
  Repeating Sequence/1 -> Switch/1
  Switch/1 -> Scope/2, Relational Operator/2
  Vref_state/1 -> Scope/3, Switch1/2, Switch/2
  Switch1/1 -> Gain2/1, Scope/1
  Vref/1 -> Switch1/1

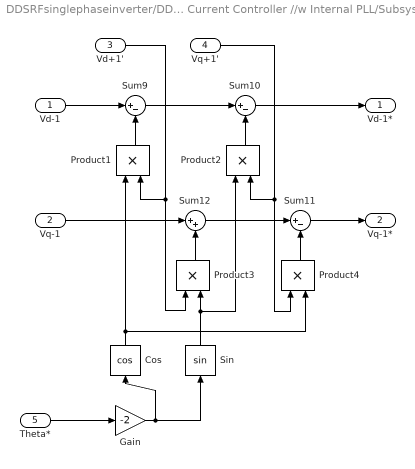
== system DDSRFsinglephaseinverter/DDSRF Current Controller //w Internal PLL/Subsystem1 ==
  Vd-1 : Inport
  Vq-1 : Inport  Port=2
  Vd+1' : Inport  Port=3
  Vq+1' : Inport  Port=4
  Theta* : Inport  Port=5
  Cos : Trigonometry  Operator=cos
  Gain : Gain  Gain=-2
  Product{1..4} (4 alike) : Product
  Sin : Trigonometry
  Sum10 : Sum  Inputs=|+-
  Sum11 : Sum  Inputs=|+-
  Sum12 : Sum  Inputs=|++
  Sum9 : Sum  Inputs=|+-
  Vd-1* : Outport
  Vq-1* : Outport  Port=2
  wires:
  Sum11/1 -> Vq-1*/1
  Sin/1 -> Product2/1, Product3/2
  Theta*/1 -> Gain/1
  Vq+1'/1 -> Product4/1, Product2/2
  Product2/1 -> Sum10/2
  Vq-1/1 -> Sum12/1
  Sum10/1 -> Vd-1*/1
  Cos/1 -> Product4/2, Product1/1
  Sum9/1 -> Sum10/1
  Product1/1 -> Sum9/2
  Product4/1 -> Sum11/2
  Gain/1 -> Sin/1, Cos/1
  Vd+1'/1 -> Product3/1, Product1/2
  Vd-1/1 -> Sum9/1
  Product3/1 -> Sum12/2
  Sum12/1 -> Sum11/1

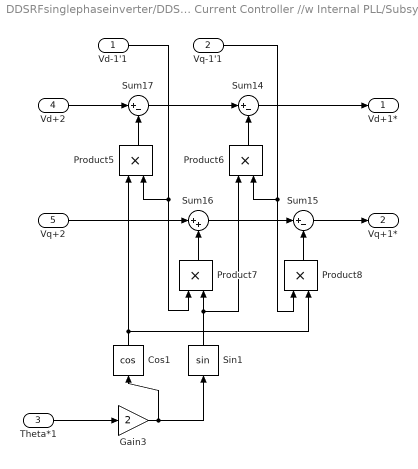
== system DDSRFsinglephaseinverter/DDSRF Current Controller //w Internal PLL/Subsystem2 ==
  Vd-1'1 : Inport
  Vq-1'1 : Inport  Port=2
  Theta*1 : Inport  Port=3
  Vd+2 : Inport  Port=4
  Vq+2 : Inport  Port=5
  Cos1 : Trigonometry  Operator=cos
  Gain3 : Gain  Gain=2
  Product{5..8} (4 alike) : Product
  Sin1 : Trigonometry
  Sum14 : Sum  Inputs=|+-
  Sum15 : Sum  Inputs=|+-
  Sum16 : Sum  Inputs=|++
  Sum17 : Sum  Inputs=|+-
  Vd+1* : Outport
  Vq+1* : Outport  Port=2
  wires:
  Cos1/1 -> Product8/2, Product5/1
  Vd+2/1 -> Sum17/1
  Vd-1'1/1 -> Product7/1, Product5/2
  Gain3/1 -> Sin1/1, Cos1/1
  Sin1/1 -> Product6/1, Product7/2
  Product5/1 -> Sum17/2
  Sum16/1 -> Sum15/1
  Sum14/1 -> Vd+1*/1
  Vq+2/1 -> Sum16/1
  Theta*1/1 -> Gain3/1
  Vq-1'1/1 -> Product8/1, Product6/2
  Product6/1 -> Sum14/2
  Sum17/1 -> Sum14/1
  Product8/1 -> Sum15/2
  Sum15/1 -> Vq+1*/1
  Product7/1 -> Sum16/2

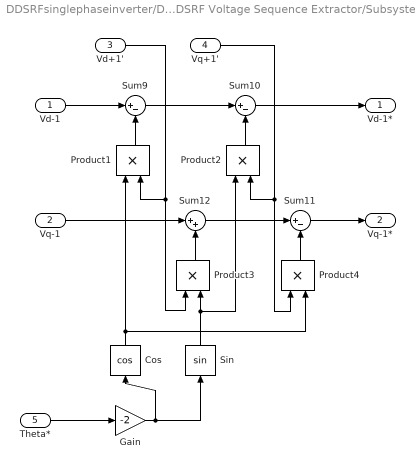
== system DDSRFsinglephaseinverter/DDSRF Voltage Sequence Extractor/Subsystem2 ==
  Vd-1 : Inport
  Vq-1 : Inport  Port=2
  Vd+1' : Inport  Port=3
  Vq+1' : Inport  Port=4
  Theta* : Inport  Port=5
  Cos : Trigonometry  Operator=cos
  Gain : Gain  Gain=-2
  Product{1..4} (4 alike) : Product
  Sin : Trigonometry
  Sum10 : Sum  Inputs=|+-
  Sum11 : Sum  Inputs=|+-
  Sum12 : Sum  Inputs=|++
  Sum9 : Sum  Inputs=|+-
  Vd-1* : Outport
  Vq-1* : Outport  Port=2
  wires:
  Sum11/1 -> Vq-1*/1
  Sin/1 -> Product2/1, Product3/2
  Theta*/1 -> Gain/1
  Vq+1'/1 -> Product4/1, Product2/2
  Product2/1 -> Sum10/2
  Vq-1/1 -> Sum12/1
  Sum10/1 -> Vd-1*/1
  Cos/1 -> Product4/2, Product1/1
  Sum9/1 -> Sum10/1
  Product1/1 -> Sum9/2
  Product4/1 -> Sum11/2
  Gain/1 -> Sin/1, Cos/1
  Vd+1'/1 -> Product3/1, Product1/2
  Vd-1/1 -> Sum9/1
  Product3/1 -> Sum12/2
  Sum12/1 -> Sum11/1

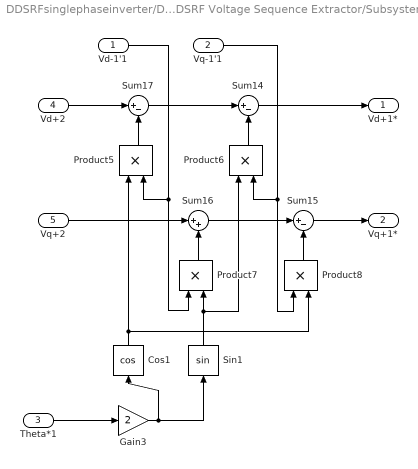
== system DDSRFsinglephaseinverter/DDSRF Voltage Sequence Extractor/Subsystem3 ==
  Vd-1'1 : Inport
  Vq-1'1 : Inport  Port=2
  Theta*1 : Inport  Port=3
  Vd+2 : Inport  Port=4
  Vq+2 : Inport  Port=5
  Cos1 : Trigonometry  Operator=cos
  Gain3 : Gain  Gain=2
  Product{5..8} (4 alike) : Product
  Sin1 : Trigonometry
  Sum14 : Sum  Inputs=|+-
  Sum15 : Sum  Inputs=|+-
  Sum16 : Sum  Inputs=|++
  Sum17 : Sum  Inputs=|+-
  Vd+1* : Outport
  Vq+1* : Outport  Port=2
  wires:
  Cos1/1 -> Product8/2, Product5/1
  Vd+2/1 -> Sum17/1
  Vd-1'1/1 -> Product7/1, Product5/2
  Gain3/1 -> Sin1/1, Cos1/1
  Sin1/1 -> Product6/1, Product7/2
  Product5/1 -> Sum17/2
  Sum16/1 -> Sum15/1
  Sum14/1 -> Vd+1*/1
  Vq+2/1 -> Sum16/1
  Theta*1/1 -> Gain3/1
  Vq-1'1/1 -> Product8/1, Product6/2
  Product6/1 -> Sum14/2
  Sum17/1 -> Sum14/1
  Product8/1 -> Sum15/2
  Sum15/1 -> Vq+1*/1
  Product7/1 -> Sum16/2
